simulink model "part12"  (R2020a)
settings: Solver=VariableStepAuto  StartTime=0.0  StopTime=40.0  RelTol=1e-3
settings Model: Creator=emami  LastModifiedBy=emami

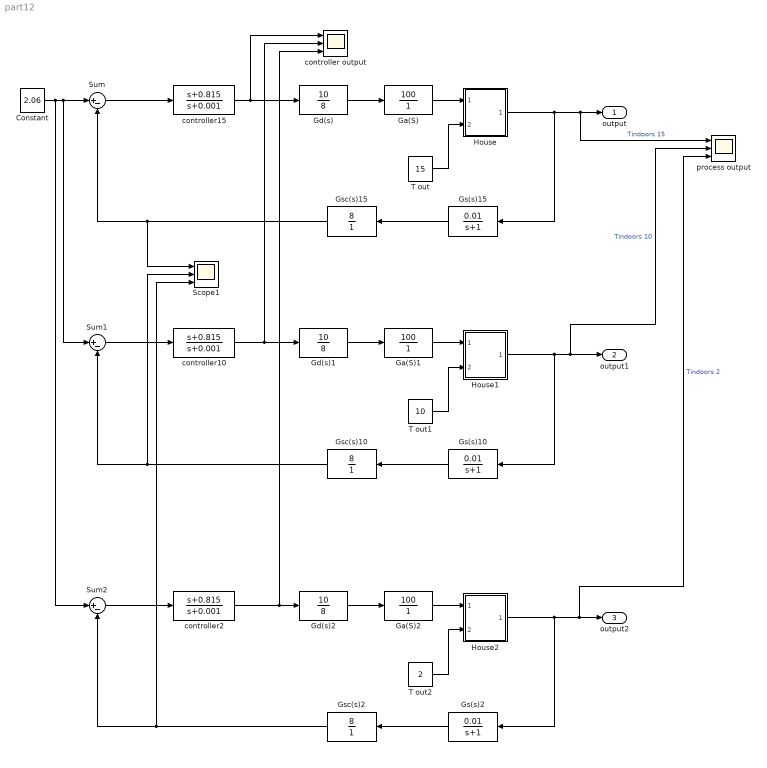
== system part12 ==
  " Gs(s)10" : TransferFcn  Numerator=[0.01]  Denominator=[1 1]
  " Gs(s)15" : TransferFcn  Numerator=[0.01]  Denominator=[1 1]
  " Gs(s)2" : TransferFcn  Numerator=[0.01]  Denominator=[1 1]
  " Gsc(s)10" : TransferFcn  Numerator=[8]  Denominator=[1]
  " Gsc(s)15" : TransferFcn  Numerator=[8]  Denominator=[1]
  " Gsc(s)2" : TransferFcn  Numerator=[8]  Denominator=[1]
  Constant : Constant  Value=2.06
  Ga(S) : TransferFcn  Numerator=[100]  Denominator=[1]
  Ga(S)1 : TransferFcn  Numerator=[100]  Denominator=[1]
  Ga(S)2 : TransferFcn  Numerator=[100]  Denominator=[1]
  Gd(s) : TransferFcn  Numerator=[10]  Denominator=[8]
  Gd(s)1 : TransferFcn  Numerator=[10]  Denominator=[8]
  Gd(s)2 : TransferFcn  Numerator=[10]  Denominator=[8]
  House : Subsystem
      mask Display: image(fullfile(matlabroot,'toolbox','simulink','simdemos','simgeneral','images','HouseHeatHousePix.svg'))
  House1 : Subsystem
      mask Display: image(fullfile(matlabroot,'toolbox','simulink','simdemos','simgeneral','images','HouseHeatHousePix.svg'))
  House2 : Subsystem
      mask Display: image(fullfile(matlabroot,'toolbox','simulink','simdemos','simgeneral','images','HouseHeatHousePix.svg'))
  Scope1 : Scope  NumInputPorts=3
  Sum : Sum  Inputs=|+-
  Sum1 : Sum  Inputs=|+-
  Sum2 : Sum  Inputs=|+-
  T out : Constant  Value=15
  T out1 : Constant  Value=10
  T out2 : Constant  Value=2
  controller output : Scope  NumInputPorts=3
  controller10 : TransferFcn  Numerator=[1 0.815]  Denominator=[1 0.001]
  controller15 : TransferFcn  Numerator=[1 0.815]  Denominator=[1 0.001]
  controller2 : TransferFcn  Numerator=[1 0.815]  Denominator=[1 0.001]
  process output : Scope  NumInputPorts=3
  output : Outport
  output1 : Outport  Port=2
  output2 : Outport  Port=3
  wires:
  Sum/1 -> controller15/1
  Gd(s)/1 -> Ga(S)/1
  " Gsc(s)15"/1 -> Scope1/1, Sum/2
  " Gs(s)15"/1 -> " Gsc(s)15"/1
  House/1(Room Temp Troom) -> " Gs(s)15"/1, process output/1, output/1  "Tindoors 15"
  T out/1 -> House/2(Outdoor Temp Tout)
  Ga(S)/1 -> House/1(Heater QDot In)
  controller15/1 -> Gd(s)/1, controller output/1
  Sum1/1 -> controller10/1
  Gd(s)1/1 -> Ga(S)1/1
  " Gsc(s)10"/1 -> Scope1/2, Sum1/2
  " Gs(s)10"/1 -> " Gsc(s)10"/1
  House1/1(Room Temp Troom) -> " Gs(s)10"/1, process output/2, output1/1  "Tindoors 10"
  T out1/1 -> House1/2(Outdoor Temp Tout)
  Ga(S)1/1 -> House1/1(Heater QDot In)
  Sum2/1 -> controller2/1
  Gd(s)2/1 -> Ga(S)2/1
  " Gsc(s)2"/1 -> Scope1/3, Sum2/2
  " Gs(s)2"/1 -> " Gsc(s)2"/1
  Constant/1 -> Sum2/1, Sum1/1, Sum/1
  House2/1(Room Temp Troom) -> " Gs(s)2"/1, process output/3, output2/1  "Tindoors 2"
  T out2/1 -> House2/2(Outdoor Temp Tout)
  Ga(S)2/1 -> House2/1(Heater QDot In)
  controller2/1 -> controller output/3, Gd(s)2/1
  controller10/1 -> controller output/2, Gd(s)1/1

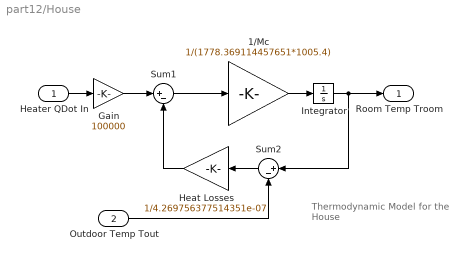
== system part12/House ==
  note: Thermodynamic Model
      | for the House
  Heater QDot In : Inport
  Outdoor Temp Tout : Inport  Port=2
  1/Mc : Gain  Gain=1/(1778.369114457651*1005.4)  SaturateOnIntegerOverflow=on  OutDataTypeStr=Inherit: Same as input  ParamDataTypeStr=Inherit: Same as input
  Gain : Gain  Gain=100000
  Heat Losses : Gain  Gain=1/4.269756377514351e-07  SaturateOnIntegerOverflow=on  OutDataTypeStr=Inherit: Same as input  ParamDataTypeStr=Inherit: Same as input
  Integrator : Integrator  InitialCondition=20
  Sum1 : Sum  Inputs=|+-  InputSameDT=on  SaturateOnIntegerOverflow=on  OutDataTypeStr=Inherit: Same as first input
  Sum2 : Sum  Inputs=|+-  InputSameDT=on  SaturateOnIntegerOverflow=on  OutDataTypeStr=Inherit: Same as first input
  Room Temp Troom : Outport  InitialOutput=0
  wires:
  Outdoor Temp Tout/1 -> Sum2/2
  Heater QDot In/1 -> Gain/1
  Sum1/1 -> 1/Mc/1
  Sum2/1 -> Heat Losses/1
  Heat Losses/1 -> Sum1/2
  1/Mc/1 -> Integrator/1
  Integrator/1 -> Sum2/1, Room Temp Troom/1
  Gain/1 -> Sum1/1

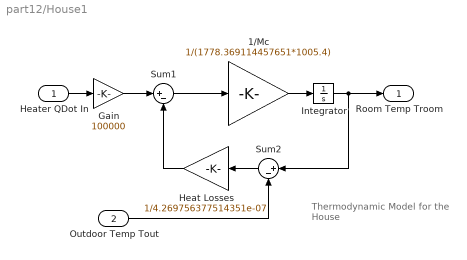
== system part12/House1 ==
  note: Thermodynamic Model
      | for the House
  Heater QDot In : Inport
  Outdoor Temp Tout : Inport  Port=2
  1/Mc : Gain  Gain=1/(1778.369114457651*1005.4)  SaturateOnIntegerOverflow=on  OutDataTypeStr=Inherit: Same as input  ParamDataTypeStr=Inherit: Same as input
  Gain : Gain  Gain=100000
  Heat Losses : Gain  Gain=1/4.269756377514351e-07  SaturateOnIntegerOverflow=on  OutDataTypeStr=Inherit: Same as input  ParamDataTypeStr=Inherit: Same as input
  Integrator : Integrator  InitialCondition=20
  Sum1 : Sum  Inputs=|+-  InputSameDT=on  SaturateOnIntegerOverflow=on  OutDataTypeStr=Inherit: Same as first input
  Sum2 : Sum  Inputs=|+-  InputSameDT=on  SaturateOnIntegerOverflow=on  OutDataTypeStr=Inherit: Same as first input
  Room Temp Troom : Outport  InitialOutput=0
  wires:
  Outdoor Temp Tout/1 -> Sum2/2
  Heater QDot In/1 -> Gain/1
  Sum1/1 -> 1/Mc/1
  Sum2/1 -> Heat Losses/1
  Heat Losses/1 -> Sum1/2
  1/Mc/1 -> Integrator/1
  Integrator/1 -> Sum2/1, Room Temp Troom/1
  Gain/1 -> Sum1/1

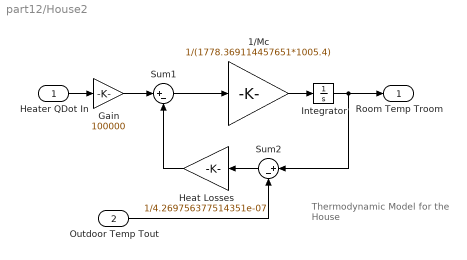
== system part12/House2 ==
  note: Thermodynamic Model
      | for the House
  Heater QDot In : Inport
  Outdoor Temp Tout : Inport  Port=2
  1/Mc : Gain  Gain=1/(1778.369114457651*1005.4)  SaturateOnIntegerOverflow=on  OutDataTypeStr=Inherit: Same as input  ParamDataTypeStr=Inherit: Same as input
  Gain : Gain  Gain=100000
  Heat Losses : Gain  Gain=1/4.269756377514351e-07  SaturateOnIntegerOverflow=on  OutDataTypeStr=Inherit: Same as input  ParamDataTypeStr=Inherit: Same as input
  Integrator : Integrator  InitialCondition=20
  Sum1 : Sum  Inputs=|+-  InputSameDT=on  SaturateOnIntegerOverflow=on  OutDataTypeStr=Inherit: Same as first input
  Sum2 : Sum  Inputs=|+-  InputSameDT=on  SaturateOnIntegerOverflow=on  OutDataTypeStr=Inherit: Same as first input
  Room Temp Troom : Outport  InitialOutput=0
  wires:
  Outdoor Temp Tout/1 -> Sum2/2
  Heater QDot In/1 -> Gain/1
  Sum1/1 -> 1/Mc/1
  Sum2/1 -> Heat Losses/1
  Heat Losses/1 -> Sum1/2
  1/Mc/1 -> Integrator/1
  Integrator/1 -> Sum2/1, Room Temp Troom/1
  Gain/1 -> Sum1/1
